simulink model "hexafinal"  (R2022b)
settings: Solver=ode8  StartTime=0.0  StopTime=6  FixedStep=0.001  RelTol=1e-3
InitFcn:
  | untitled2
values from neighbouring files (symbols this model uses):
  alph1 = 21    [untitled2.m]
  alph2 = 146    [untitled2.m]
  alph3 = 336    [untitled2.m]
  g = 9.8    [untitled2.m]
  J = diag([0.0820,0.0845,0.1377])    [untitled2.m]
  J_inv = inv(J)    [untitled2.m]
  k = 30    [untitled2.m]
  k_omega = ( J_inv )*( 2.54 )    [untitled2.m]
  k_omega_smc = 0.10*( J_inv )*( 16 )    [untitled2.m]
  k_R = ( J_inv )*( 8.81 )    [untitled2.m]
  k_R_smc = 0.25*( J_inv )*( 20 )    [untitled2.m]
  k_v = 22    [untitled2.m]
  k_x = 35    [untitled2.m]
  kappa = 50    [untitled2.m]
  l = [   0.05 ... (first row only)    [untitled2.m]
  lv = [ 0.5 ... (first row only)    [untitled2.m]
  m = 4.34    [untitled2.m]
undefined symbols (not defined in the file or in its folder): normc
settings Model: Creator=edgar  LastModifiedBy=gerar
settings SolverCC: ZeroCrossAlgorithm=Adaptive  AlgebraicLoopSolver=LineSearch
settings DebuggingCC: IgnoredZcDiagnostic=none  UnconnectedInputMsg=warning  UnconnectedOutputMsg=warning  UnconnectedLineMsg=warning  SFMachineParentedDataDiag=warning
settings ModelReferenceCC: EnableRefExpFcnMdlSchedulingChecks=on
settings SFSimCC: CustomCodeUndefinedFunction=UseInterfaceOnly

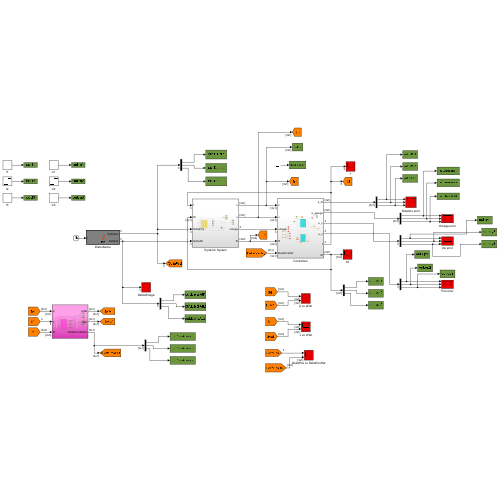
[thumbnail: Simulink's stored preview of the top-level diagram]
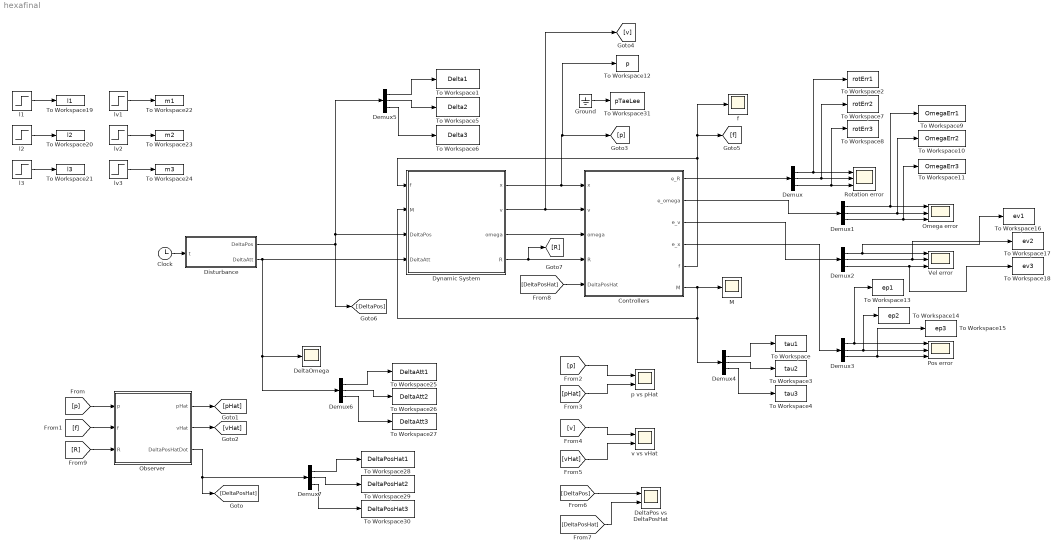
== system hexafinal ==
  Clock : Clock
  Controllers : Subsystem
  DeltaOmega : Scope
  DeltaPos vs DeltaPosHat : Scope  NumInputPorts=2
  Demux{,1..7} (8 alike) : Demux  Outputs=3
  Disturbance : MATLAB Function  TreatAsAtomicUnit=on
  "Dynamic System " : Subsystem
  Ground : Ground
  M : Scope
  Observer : Subsystem
  "Omega error " : Scope  NumInputPorts=3
  Pos error : Scope  NumInputPorts=3
  "Rotation error " : Scope  NumInputPorts=3
  To Workspace : ToWorkspace  VariableName=tau1  SaveFormat=Timeseries  SampleTime=-1
  To Workspace1 : ToWorkspace  VariableName=Delta1  SaveFormat=Timeseries  SampleTime=-1
  To Workspace10 : ToWorkspace  VariableName=OmegaErr2  SaveFormat=Timeseries  SampleTime=-1
  To Workspace11 : ToWorkspace  VariableName=OmegaErr3  SaveFormat=Timeseries  SampleTime=-1
  To Workspace12 : ToWorkspace  VariableName=p  SampleTime=-1
  To Workspace13 : ToWorkspace  VariableName=ep1  SaveFormat=Timeseries  SampleTime=-1
  To Workspace14 : ToWorkspace  VariableName=ep2  SaveFormat=Timeseries  SampleTime=-1
  To Workspace15 : ToWorkspace  VariableName=ep3  SaveFormat=Timeseries  SampleTime=-1
  To Workspace16 : ToWorkspace  VariableName=ev1  SaveFormat=Timeseries  SampleTime=-1
  To Workspace17 : ToWorkspace  VariableName=ev2  SaveFormat=Timeseries  SampleTime=-1
  To Workspace18 : ToWorkspace  VariableName=ev3  SaveFormat=Timeseries  SampleTime=-1
  To Workspace19 : ToWorkspace  VariableName=l1  SaveFormat=Timeseries  SampleTime=-1
  To Workspace2 : ToWorkspace  VariableName=rotErr1  SaveFormat=Timeseries  SampleTime=-1
  To Workspace20 : ToWorkspace  VariableName=l2  SaveFormat=Timeseries  SampleTime=-1
  To Workspace21 : ToWorkspace  VariableName=l3  SaveFormat=Timeseries  SampleTime=-1
  To Workspace22 : ToWorkspace  VariableName=m1  SaveFormat=Timeseries  SampleTime=-1
  To Workspace23 : ToWorkspace  VariableName=m2  SaveFormat=Timeseries  SampleTime=-1
  To Workspace24 : ToWorkspace  VariableName=m3  SaveFormat=Timeseries  SampleTime=-1
  To Workspace25 : ToWorkspace  VariableName=DeltaAtt1  SaveFormat=Timeseries  SampleTime=-1
  To Workspace26 : ToWorkspace  VariableName=DeltaAtt2  SaveFormat=Timeseries  SampleTime=-1
  To Workspace27 : ToWorkspace  VariableName=DeltaAtt3  SaveFormat=Timeseries  SampleTime=-1
  To Workspace28 : ToWorkspace  VariableName=DeltaPosHat1  SaveFormat=Timeseries  SampleTime=-1
  To Workspace29 : ToWorkspace  VariableName=DeltaPosHat2  SaveFormat=Timeseries  SampleTime=-1
  To Workspace3 : ToWorkspace  VariableName=tau2  SaveFormat=Timeseries  SampleTime=-1
  To Workspace30 : ToWorkspace  VariableName=DeltaPosHat3  SaveFormat=Timeseries  SampleTime=-1
  To Workspace31 : ToWorkspace  VariableName=pTaeLee  SampleTime=-1
  To Workspace4 : ToWorkspace  VariableName=tau3  SaveFormat=Timeseries  SampleTime=-1
  To Workspace5 : ToWorkspace  VariableName=Delta2  SaveFormat=Timeseries  SampleTime=-1
  To Workspace6 : ToWorkspace  VariableName=Delta3  SaveFormat=Timeseries  SampleTime=-1
  To Workspace7 : ToWorkspace  VariableName=rotErr2  SaveFormat=Timeseries  SampleTime=-1
  To Workspace8 : ToWorkspace  VariableName=rotErr3  SaveFormat=Timeseries  SampleTime=-1
  To Workspace9 : ToWorkspace  VariableName=OmegaErr1  SaveFormat=Timeseries  SampleTime=-1
  Vel error : Scope  NumInputPorts=3
  f : Scope
  l1 : Step  Time=0  Before=l(1,1)  After=l(1,1)  SampleTime=0
  l2 : Step  Time=0  Before=l(2,1)  After=l(2,1)  SampleTime=0
  l3 : Step  Time=0  Before=l(3,1)  After=l(3,1)  SampleTime=0
  lv1 : Step  Time=0  Before=lv(1,1)  After=lv(1,1)  SampleTime=0
  lv2 : Step  Time=0  Before=lv(2,1)  After=lv(2,1)  SampleTime=0
  lv3 : Step  Time=0  Before=lv(3,1)  After=lv(3,1)  SampleTime=0
  p vs pHat : Scope  NumInputPorts=2
  v vs vHat : Scope  NumInputPorts=2
  wires:
  Demux/1 -> "Rotation error "/1, To Workspace2/1
  Demux/2 -> "Rotation error "/2, To Workspace7/1
  Demux/3 -> "Rotation error "/3, To Workspace8/1
  Demux1/1 -> To Workspace9/1, "Omega error "/1
  Demux1/2 -> To Workspace10/1, "Omega error "/2
  Demux1/3 -> To Workspace11/1, "Omega error "/3
  Controllers/1(e_R) -> Demux/1
  Controllers/2(e_omega) -> Demux1/1
  Demux2/1 -> To Workspace16/1, Vel error/1
  Demux2/2 -> To Workspace17/1, Vel error/2
  Demux2/3 -> To Workspace18/1, Vel error/3
  Controllers/3(e_v) -> Demux2/1
  "Dynamic System "/1(x) -> To Workspace12/1, [p], Controllers/1(x)
  "Dynamic System "/2(v) -> [v], Controllers/2(v)
  "Dynamic System "/3(omega) -> Controllers/3(omega)
  Demux3/3 -> To Workspace15/1, Pos error/3
  Controllers/4(e_x) -> Demux3/1
  Demux3/1 -> To Workspace13/1, Pos error/1
  Demux3/2 -> Pos error/2, To Workspace14/1
  Controllers/5(f) -> f/1, [f], "Dynamic System "/1(f)
  Controllers/6(M) -> M/1, Demux4/1, "Dynamic System "/2(M)
  Clock/1 -> Disturbance/1(t)
  Disturbance/1(DeltaPos) -> [DeltaPos], "Dynamic System "/3(DeltaPos), Demux5/1
  Demux4/1 -> To Workspace/1
  Demux4/2 -> To Workspace3/1
  Demux4/3 -> To Workspace4/1
  Demux5/1 -> To Workspace1/1
  Demux5/2 -> To Workspace5/1
  Demux5/3 -> To Workspace6/1
  Observer/2(vHat) -> [vHat]
  [DeltaPosHat] -> DeltaPos vs DeltaPosHat/2
  [p] -> p vs pHat/1
  [p] -> Observer/1(p)
  [vHat] -> v vs vHat/2
  [v] -> v vs vHat/1
  Observer/1(pHat) -> [pHat]
  [pHat] -> p vs pHat/2
  Observer/3(DeltaPosHatDot) -> Demux7/1, [DeltaPosHat]
  [f] -> Observer/2(f)
  [DeltaPos] -> DeltaPos vs DeltaPosHat/1
  [DeltaPosHat] -> Controllers/5(DeltaPosHat)
  [R] -> Observer/3(R)
  Disturbance/2(DeltaAtt) -> DeltaOmega/1, Demux6/1, "Dynamic System "/4(DeltaAtt)
  l1/1 -> To Workspace19/1
  l2/1 -> To Workspace20/1
  l3/1 -> To Workspace21/1
  lv1/1 -> To Workspace22/1
  lv2/1 -> To Workspace23/1
  lv3/1 -> To Workspace24/1
  Demux6/3 -> To Workspace27/1
  Demux6/2 -> To Workspace26/1
  Demux6/1 -> To Workspace25/1
  Demux7/2 -> To Workspace29/1
  Demux7/1 -> To Workspace28/1
  Demux7/3 -> To Workspace30/1
  "Dynamic System "/4(R) -> [R], Controllers/4(R)
  Ground/1 -> To Workspace31/1

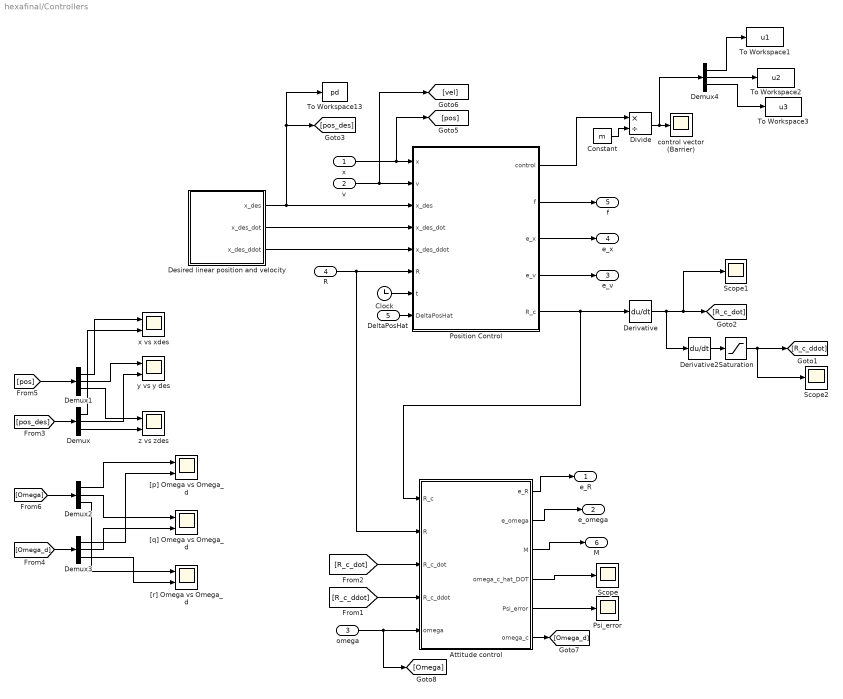
== system hexafinal/Controllers ==
  x : Inport
  v : Inport  Port=2
  omega : Inport  Port=3
  R : Inport  Port=4
  DeltaPosHat : Inport  Port=5
  Attitude control : MATLAB Function  TreatAsAtomicUnit=on
  Clock : Clock
  Constant : Constant  Value=m
  Demux{,1..4} (5 alike) : Demux  Outputs=3
  Derivative : Derivative
  Derivative2 : Derivative
  Desired linear position and velocity : Subsystem
  Divide : Product  Inputs=*/
  Position Control : MATLAB Function  TreatAsAtomicUnit=on
  Psi_error : Scope
  Saturation : Saturate  UpperLimit=30  LowerLimit=-30
  Scope : Scope
  Scope1 : Scope
  Scope2 : Scope
  To Workspace1 : ToWorkspace  VariableName=u1  SaveFormat=Timeseries  SampleTime=-1
  To Workspace13 : ToWorkspace  VariableName=pd  SampleTime=-1
  To Workspace2 : ToWorkspace  VariableName=u2  SaveFormat=Timeseries  SampleTime=-1
  To Workspace3 : ToWorkspace  VariableName=u3  SaveFormat=Timeseries  SampleTime=-1
  "[p] Omega vs Omega_d" : Scope  NumInputPorts=2
  "[q] Omega vs Omega_d" : Scope  NumInputPorts=2
  "[r] Omega vs Omega_d" : Scope  NumInputPorts=2
  control vector (Barrier) : Scope
  x vs xdes : Scope  NumInputPorts=2
  y vs y des : Scope  NumInputPorts=2
  z vs zdes : Scope  NumInputPorts=2
  e_R : Outport
  e_omega : Outport  Port=2
  e_v : Outport  Port=3
  e_x : Outport  Port=4
  f : Outport  Port=5
  M : Outport  Port=6
  wires:
  Desired linear position and velocity/2(x_des_dot) -> Position Control/4(x_des_dot)
  Desired linear position and velocity/1(x_des) -> To Workspace13/1, [pos_des], Position Control/3(x_des)
  x/1 -> [pos], Position Control/1(x)
  v/1 -> [vel], Position Control/2(v)
  R/1 -> Position Control/6(R), Attitude control/2(R)
  Position Control/2(f) -> f/1
  Desired linear position and velocity/3(x_des_ddot) -> Position Control/5(x_des_ddot)
  Position Control/5(R_c) -> Attitude control/1(R_c), Derivative/1
  Derivative/1 -> Derivative2/1, Scope1/1, [R_c_dot]
  [R_c_dot] -> Attitude control/3(R_c_dot)
  omega/1 -> [Omega], Attitude control/5(omega)
  Attitude control/1(e_R) -> e_R/1
  Attitude control/2(e_omega) -> e_omega/1
  Position Control/3(e_x) -> e_x/1
  Position Control/4(e_v) -> e_v/1
  Attitude control/3(M) -> M/1
  Derivative2/1 -> Saturation/1
  [R_c_ddot] -> Attitude control/4(R_c_ddot)
  Attitude control/4(omega_c_hat_DOT) -> Scope/1
  Clock/1 -> Position Control/7(t)
  Attitude control/5(Psi_error) -> Psi_error/1
  [pos_des] -> Demux/1
  [pos] -> Demux1/1
  [Omega] -> Demux2/1
  [Omega_d] -> Demux3/1
  Demux1/1 -> x vs xdes/1
  Demux/1 -> x vs xdes/2
  Demux1/2 -> y vs y des/1
  Demux/2 -> y vs y des/2
  Demux1/3 -> z vs zdes/1
  Demux/3 -> z vs zdes/2
  Attitude control/6(omega_c) -> [Omega_d]
  Demux3/1 -> "[p] Omega vs Omega_d"/2
  Demux2/1 -> "[p] Omega vs Omega_d"/1
  Demux2/2 -> "[q] Omega vs Omega_d"/1
  Demux3/2 -> "[q] Omega vs Omega_d"/2
  Demux2/3 -> "[r] Omega vs Omega_d"/1
  Demux3/3 -> "[r] Omega vs Omega_d"/2
  Saturation/1 -> Scope2/1, [R_c_ddot]
  DeltaPosHat/1 -> Position Control/8(DeltaPosHat)
  Divide/1 -> Demux4/1, control vector (Barrier)/1
  Position Control/1(control) -> Divide/1
  Constant/1 -> Divide/2
  Demux4/1 -> To Workspace1/1
  Demux4/2 -> To Workspace2/1
  Demux4/3 -> To Workspace3/1

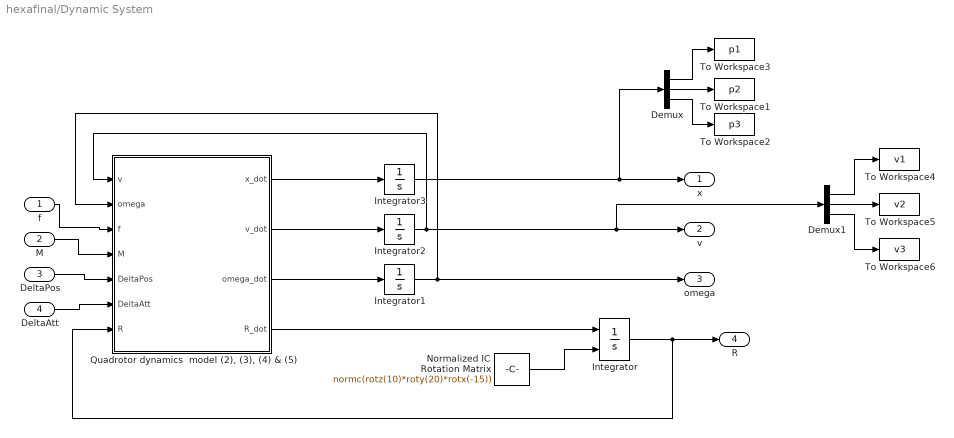
== system hexafinal/Dynamic System  ==
  f : Inport
  M : Inport  Port=2
  DeltaPos : Inport  Port=3
  DeltaAtt : Inport  Port=4
  Demux : Demux  Outputs=3
  Demux1 : Demux  Outputs=3
  Integrator : Integrator  InitialConditionSource=external  InitialCondition=eye(3)
  Integrator1 : Integrator  InitialCondition=[0;0;0]
  Integrator2 : Integrator  InitialCondition=[0;0;0]
  Integrator3 : Integrator  InitialCondition=[0;0;0]
  "Normalized IC Rotation Matrix " : Constant  Value=normc(rotz(10)*roty(20)*rotx(-15))
  "Quadrotor dynamics  model (2), (3), (4) & (5)" : MATLAB Function  TreatAsAtomicUnit=on
  To Workspace1 : ToWorkspace  VariableName=p2  SaveFormat=Timeseries  SampleTime=-1
  To Workspace2 : ToWorkspace  VariableName=p3  SaveFormat=Timeseries  SampleTime=-1
  To Workspace3 : ToWorkspace  VariableName=p1  SaveFormat=Timeseries  SampleTime=-1
  To Workspace4 : ToWorkspace  VariableName=v1  SaveFormat=Timeseries  SampleTime=-1
  To Workspace5 : ToWorkspace  VariableName=v2  SaveFormat=Timeseries  SampleTime=-1
  To Workspace6 : ToWorkspace  VariableName=v3  SaveFormat=Timeseries  SampleTime=-1
  x : Outport
  v : Outport  Port=2
  omega : Outport  Port=3
  R : Outport  Port=4
  wires:
  Integrator3/1 -> Demux/1, x/1
  "Quadrotor dynamics  model (2), (3), (4) & (5)"/3(omega_dot) -> Integrator1/1
  "Quadrotor dynamics  model (2), (3), (4) & (5)"/1(x_dot) -> Integrator3/1
  "Quadrotor dynamics  model (2), (3), (4) & (5)"/2(v_dot) -> Integrator2/1
  Integrator/1 -> R/1, "Quadrotor dynamics  model (2), (3), (4) & (5)"/7(R)
  "Quadrotor dynamics  model (2), (3), (4) & (5)"/4(R_dot) -> Integrator/1
  Integrator1/1 -> omega/1, "Quadrotor dynamics  model (2), (3), (4) & (5)"/2(omega)
  Integrator2/1 -> Demux1/1, v/1, "Quadrotor dynamics  model (2), (3), (4) & (5)"/1(v)
  f/1 -> "Quadrotor dynamics  model (2), (3), (4) & (5)"/3(f)
  M/1 -> "Quadrotor dynamics  model (2), (3), (4) & (5)"/4(M)
  "Normalized IC Rotation Matrix "/1 -> Integrator/2
  DeltaPos/1 -> "Quadrotor dynamics  model (2), (3), (4) & (5)"/5(DeltaPos)
  DeltaAtt/1 -> "Quadrotor dynamics  model (2), (3), (4) & (5)"/6(DeltaAtt)
  Demux1/1 -> To Workspace4/1
  Demux1/2 -> To Workspace5/1
  Demux1/3 -> To Workspace6/1
  Demux/1 -> To Workspace3/1
  Demux/2 -> To Workspace1/1
  Demux/3 -> To Workspace2/1

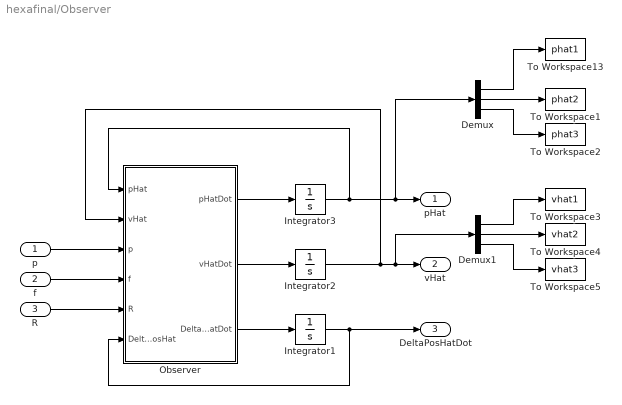
== system hexafinal/Observer ==
  p : Inport
  f : Inport  Port=2
  R : Inport  Port=3
  Demux : Demux  Outputs=3
  Demux1 : Demux  Outputs=3
  Integrator1 : Integrator  InitialCondition=[0;0;0]
  Integrator2 : Integrator  InitialCondition=[0;0;0]
  Integrator3 : Integrator  InitialCondition=[0;0;0]
  Observer : MATLAB Function  TreatAsAtomicUnit=on
  To Workspace1 : ToWorkspace  VariableName=phat2  SaveFormat=Timeseries  SampleTime=-1
  To Workspace13 : ToWorkspace  VariableName=phat1  SaveFormat=Timeseries  SampleTime=-1
  To Workspace2 : ToWorkspace  VariableName=phat3  SaveFormat=Timeseries  SampleTime=-1
  To Workspace3 : ToWorkspace  VariableName=vhat1  SaveFormat=Timeseries  SampleTime=-1
  To Workspace4 : ToWorkspace  VariableName=vhat2  SaveFormat=Timeseries  SampleTime=-1
  To Workspace5 : ToWorkspace  VariableName=vhat3  SaveFormat=Timeseries  SampleTime=-1
  pHat : Outport
  vHat : Outport  Port=2
  DeltaPosHatDot : Outport  Port=3
  wires:
  p/1 -> Observer/3(p)
  Observer/1(pHatDot) -> Integrator3/1
  Observer/2(vHatDot) -> Integrator2/1
  Observer/3(DeltaPosHatDot) -> Integrator1/1
  Integrator1/1 -> DeltaPosHatDot/1, Observer/6(DeltaPosHat)
  Integrator3/1 -> Observer/1(pHat), Demux/1, pHat/1
  Integrator2/1 -> Observer/2(vHat), Demux1/1, vHat/1
  f/1 -> Observer/4(f)
  R/1 -> Observer/5(R)
  Demux/1 -> To Workspace13/1
  Demux/2 -> To Workspace1/1
  Demux/3 -> To Workspace2/1
  Demux1/1 -> To Workspace3/1
  Demux1/2 -> To Workspace4/1
  Demux1/3 -> To Workspace5/1

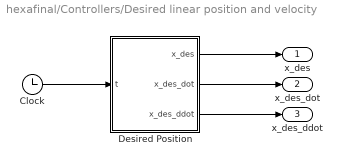
== system hexafinal/Controllers/Desired linear position and velocity ==
  Clock : Clock
  Desired Position : MATLAB Function  TreatAsAtomicUnit=on
  x_des : Outport
  x_des_dot : Outport  Port=2
  x_des_ddot : Outport  Port=3
  wires:
  Desired Position/1(x_des) -> x_des/1
  Clock/1 -> Desired Position/1(t)
  Desired Position/2(x_des_dot) -> x_des_dot/1
  Desired Position/3(x_des_ddot) -> x_des_ddot/1

== matlab function hexafinal/Controllers/Desired linear position and velocity/Desired Position ==
  data: t input; x_des output; x_des_dot output; x_des_ddot output
function [x_des, x_des_dot, x_des_ddot] = fcn(t)

%Trayectorias de Taeyung Lee; https://ieeexplore.ieee.org/stamp/stamp.jsp?arnumber=5717652
x_des     = [             0.4*t ; % 4
                  0.4*sin(pi*t) ; % 0.4
                 -0.6*cos(pi*t)]; % 0.6

x_des_dot = [               0.4 ; % 4
                0.4*pi*cos(pi*t); % 0.4*pi = 1.256
                0.6*pi*sin(pi*t)];% 0.6*pi = 1.88


x_des_ddot = [                0 ; 
            -0.4*pi^2*sin(pi*t) ; 
             0.6*pi^2*cos(pi*t)];

== matlab function hexafinal/Controllers/Attitude control ==
  data: R_c input; R input size=[3 3]; R_c_dot input; R_c_ddot input; e_R output size=[3 1]; e_omega output size=[3 1]; M output size=[3 1]; omega input size=[3 1]; J parameter; k_R parameter; k_omega parameter; omega_c_hat_DOT output; Psi_error output; omega_c output; k_R_smc parameter; k_omega_smc parameter
function [ e_R, e_omega, M, omega_c_hat_DOT, Psi_error, omega_c ] = fcn(R_c, R, R_c_dot, R_c_ddot, omega, J, k_R, k_omega, k_R_smc, k_omega_smc ) %omega_c_dot

omega_c_hat =  R_c' * R_c_dot ;           %(22)
omega_c_hat_DOT = R_c_dot'*R_c_dot + R_c'*R_c_ddot;
omega_c_DOT = [omega_c_hat_DOT(3,2); - omega_c_hat_DOT(3,1); omega_c_hat_DOT(2,1)];

omega_c = [omega_c_hat(3,2); - omega_c_hat(3,1); omega_c_hat(2,1)];



omega_hat = [0, -omega(3), omega(2);
             omega(3), 0, -omega(1);
            -omega(2), omega(1), 0];
        
R_mul = (R_c'*R) - (R'*R_c);
R_mul_vect = [R_mul(3,2); -R_mul(3,1); R_mul(2,1)];
e_R = 0.5 * R_mul_vect;   %(21)   

e_omega = omega - (R'*R_c*omega_c);  %(21)

%M = (-k_R*e_R) - (k_omega*e_omega) + cross(omega, J*omega) - J*( omega_hat*R'*R_c*omega_c - R'*R_c*omega_c_dot );  %(20)


%Proposed control for the french people
Smc_pos =  k_R_smc * [sign(e_R(1))*abs(e_R(1))^(1/2) ; 
                      sign(e_R(2))*abs(e_R(2))^(1/2) ; 
                      sign(e_R(3))*abs(e_R(3))^(1/2) ];

Smc_vel =  k_omega_smc * [  sign(e_omega(1))*abs(e_omega(1))^(1/2) ; 
                            sign(e_omega(2))*abs(e_omega(2))^(1/2) ; 
                            sign(e_omega(3))*abs(e_omega(3))^(1/2) ];

% IEEE LCSS
M =   - k_R*e_R  -  k_omega*e_omega + cross(omega, J*omega) - 1*Smc_pos - 0.1*Smc_vel - J*( omega_hat*R'*R_c*omega_c - 1*R'*R_c*omega_c_DOT ) ; 


% Taeyoung Lee controller
% M =  - k_R*e_R  - k_omega*e_omega + cross(omega, J*omega) - J*( omega_hat*R'*R_c*omega_c - R'*R_c*omega_c_DOT ) ;  %(20)

Psi_error = 1/2*trace(eye(3) - R_c'*R);

== matlab function hexafinal/Disturbance ==
  data: t input; DeltaPos output; DeltaAtt output
function [DeltaPos, DeltaAtt] = fcn(t)

%parameters
kapa1 = 1.8;
kapa2 = 1.5;
kapa3 = 1.4;




% Position distirbance
DeltaPos = [ kapa1*sin(t);                               % heaviside(t) %kapa1*sin(t);
             40*rectpuls(t-3,1) - 40*rectpuls(t-4,1);      %kapa2*cos(t)
             kapa3      ];


% Attitude distirbance
DeltaAtt = [ 1.8*cos(t); 
             0.5*sin(t) + 0.5;
             2.3*sin(t)];

== matlab function hexafinal/Observer/Observer ==
  data: pHat input; vHat input; p input; pHatDot output; vHatDot output; f input; R input; DeltaPosHat input; g parameter; m parameter; e3 parameter; alph1 parameter; alph2 parameter; alph3 parameter; eps parameter; DeltaPosHatDot output
function [pHatDot, vHatDot, DeltaPosHatDot] = obs(pHat, vHat, p, f, R, DeltaPosHat, g, m, e3, alph1, alph2, alph3, eps)

% function [pHatDot, vHatDot, omegaHatDot, RHatDot] = obs(p, vHat, omegaHat, f, M, DeltaHat, R, J_inv, J, e3, m, g)
%
% omega_hat = [           0,   - omegaHat(3),    omegaHat(2);
%              omegaHat(3),               0,  - omegaHat(1);
%            - omegaHat(2),     omegaHat(1),             0];

%      Position
pHatDot = vHat + (alph1/eps)*(p - pHat);                      
%mvHatDot = m*g*e3 - f*R*e3 + DeltaPosHat + (alph2/eps^2)*(p - pHat);  % Conventional multi-rotor
mvHatDot = m*g*e3 - R*f + DeltaPosHat + (alph2/eps^2)*(p - pHat);  % Fully-actuated multi-rotor
vHatDot = mvHatDot/m ;
DeltaPosHatDot = (alph3/eps^3)*(p - pHat);

%      Attitude
%R_dot = R * omega_hat;  %(4)
%JomDot = M - cross(omega, J*omega) + Delta;
%omega_dot = J_inv * JomDot;

== matlab function hexafinal/Controllers/Position Control ==
  data: control output; f output; e_x output; e_v output; R_c output; x input; v input size=[3 1]; x_des input size=[3 1]; x_des_dot input; x_des_ddot input; R input size=[3 3]; t input; DeltaPosHat input; k_v parameter; m parameter; g parameter; e3 parameter; k_x parameter; kappa parameter; lv parameter; l parameter; k parameter
function [control, f, e_x, e_v, R_c] = fcn( x, v, x_des, x_des_dot, x_des_ddot, R, t, DeltaPosHat, k_v, m, g, e3, k_x, kappa, lv, l, k)

e_x = x - x_des;   %(17)
e_v = v - x_des_dot;   %(18)

b1_des = [  cos(pi*t) ;  
            sin(pi*t) ;
                   0] ;

%*-*-*-*-*-*-*-*-*-*-*-*-*-*-*-*-*-*-*-*-*-*-*-*-*-*-*-*-*-*-*-*-*-*-*-*-
% Barrier control
%system errors
ep = e_x;
ev = e_v;

%backstepping errors
epsilon = ep;

%intermediate variable alpha
alpha = [ - (l(1,1)^2 - epsilon(1,1)^2) * ( k*epsilon(1,1) )  ;
          - (l(2,1)^2 - epsilon(2,1)^2) * ( k*epsilon(2,1) )  ;
          - (l(3,1)^2 - epsilon(3,1)^2) * ( k*epsilon(3,1) ) ];


zeta = ev - alpha;
alphadot = [ (k) * (3*epsilon(1,1)^2 - l(1,1)^2) * ( zeta(1,1) - ( l(1,1)^2 - epsilon(1,1)^2 )*( k*epsilon(1,1) ) )  ;
             (k) * (3*epsilon(2,1)^2 - l(2,1)^2) * ( zeta(2,1) - ( l(2,1)^2 - epsilon(2,1)^2 )*( k*epsilon(2,1) ) )  ;
             (k) * (3*epsilon(3,1)^2 - l(3,1)^2) * ( zeta(3,1) - ( l(3,1)^2 - epsilon(3,1)^2 )*( k*epsilon(3,1) ) ) ];


%control
%u = - Delta + vddot + alphadot - kappa * zeta - (epsilon)/( l^2 - epsilon^2 ) ;
%u =  - Delta + vddot + alphadot - kappa * zeta - (epsilon)/( l^2 - epsilon^2 ) - (zeta*ev)/( lv^2 - ev^2 ) - 1*(alpha) - 0*alpha^2*ev + 0*alpha^2*zeta + 0*alpha*zeta - 0*(alpha*zeta)/(lv^2 - ev^2);

%ESTE ES EL QUE DEBO PROGRAMAR [CREO QUITANDOLE ev]:
%u =  - Delta + vddot + alphadot - kappa * zeta - (epsilon)/( l^2 - epsilon^2 ) - (4*ev)/( lv^2 - ev^2 ) + 8*alpha + 8*ev;
% u = min(15, max(-15, ctrl));


logaTerms_pos = [ (epsilon(1,1))/( l(1,1)^2 - epsilon(1,1)^2 )  ;
                  (epsilon(2,1))/( l(2,1)^2 - epsilon(2,1)^2 )  ;
                  (epsilon(3,1))/( l(3,1)^2 - epsilon(3,1)^2 ) ];

logaTerms_vel = [ (4*ev(1,1))/( lv(1,1)^2 - ev(1,1)^2 )  ;
                  (4*ev(2,1))/( lv(2,1)^2 - ev(2,1)^2 )  ;
                  (4*ev(3,1))/( lv(3,1)^2 - ev(3,1)^2 ) ];

control = - m*g*e3 + m*x_des_ddot - DeltaPosHat + alphadot - kappa * zeta - logaTerms_pos - logaTerms_vel + 0.5*alpha;
%el termino - (ev)/( lv^2 - ev^2 ) hace que tambien se acote la velocidad
%[NOTE que no es el estado zeta, sino ev]

%% Fully actuated multi-rotor control:
R_c = eye(3);
f = - control;

% %% Conventional multi-rotor control:
% f = - dot( ( control ), R*e3);     %(19)
% 
% %%computed Omega & Rotation
% aa  = norm( control  );
% b3_c =  - ( control  ) / aa ;     %(23)
% 
% a1 = cross( b3_c, b1_des );
% a3 = norm( a1 );
% 
% b1_c = - ( cross(b3_c, a1) ) / a3; %(38)
% 
% a4 = cross(b3_c, b1_c);
% R_c = [b1_c  a4  b3_c];  % (22)

%*-*-*-*-*-*-*-*-*-*-*-*-*-*-*-*-*-*-*-*-*-*-*-*-*-*-*-*-*-*-*-*-*-*-*-*-

% C O M P A R I S O N  

% %Taeyung Lee control
% R_c = eye(3); % this is for the case of fully-actuated multi-rotor
% control = - m*g*e3 + m*x_des_ddot - k_x*e_x - k_v*e_v;
% f = - control;     %(19) for fully-actuated ulti-rotors
% % f = - dot( ( control) , R*e3);     %(19) for conventional multi-rotors

%Nonlinear controller for de position controlled flight mode (19) & (20)
%El mio
%f = norm(  m*g*e3 - m*x_des_ddot + k_x*e_x + k_v*e_v  );

== matlab function hexafinal/Dynamic System /Quadrotor dynamics  model (2), (3), (4) & (5) ==
  data: v input size=[3 1]; omega input; f input; x_dot output size=[3 1]; v_dot output size=[3 1]; omega_dot output; R_dot output; M input; DeltaPos input; DeltaAtt input; R input; J_inv parameter; J parameter; e3 parameter; m parameter; g parameter
function [x_dot, v_dot, omega_dot, R_dot]= fcn(v, omega, f, M, DeltaPos, DeltaAtt, R, J_inv, J, e3, m, g)

omega_hat = [0, -omega(3), omega(2);
             omega(3), 0, -omega(1);
            -omega(2), omega(1), 0];

% Position
x_dot = v;                          % (2)
%mvDot = m*g*e3 - f;                 % "f" ahora es un vector completo, sin acoplamiento
%mvDot = m*g*e3 - f*R*e3 + DeltaPos; %  Conventional multi-rotor
mvDot = m*g*e3 - R*f + DeltaPos; %  Fully actuated multi-rotor 
v_dot = mvDot/m ;

% Attitude
R_dot = R * omega_hat;  %(4)
JomDot = M - cross(omega, J*omega) + 1*DeltaAtt ; 
omega_dot = J_inv * JomDot;

%
% omega_dot = J_inv * (M - cross(omega, J*omega)  ) + J_inv * Delta; %J_inv es grande, asi que la pert es mas grande de lo que se cree
